simulink model "First_order_integrator_method"  (R2024a)
settings: Solver=VariableStepAuto  StartTime=0.0  StopTime=10.0  RelTol=1e-3
values from neighbouring files (symbols this model uses):
  b = 10    [First_order_parameters.mat]
  k = 400    [First_order_parameters.mat]
  m = 3.6    [First_order_parameters.mat]
settings Model: Creator=nassa  LastModifiedBy=nassa

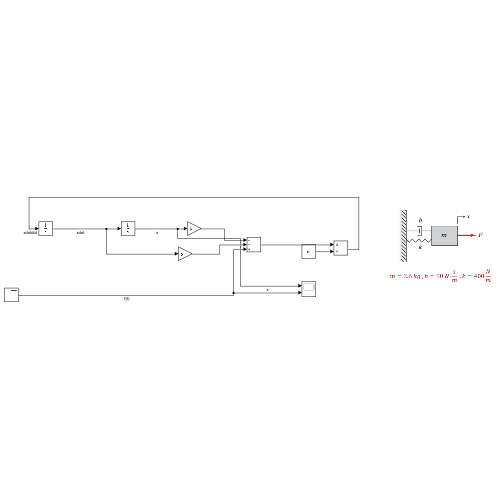
[thumbnail: Simulink's stored preview of the top-level diagram]
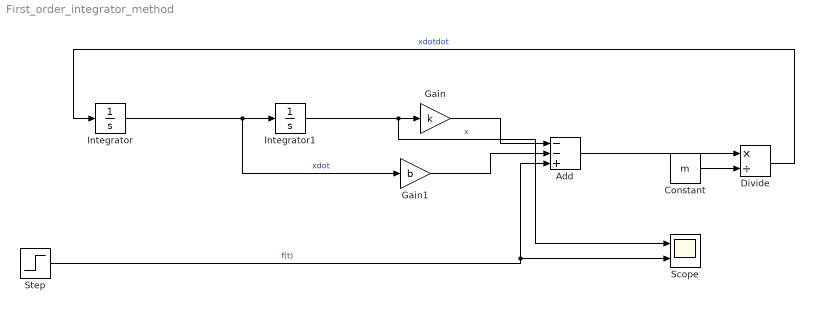
== system First_order_integrator_method ==
  Add : Sum  Inputs=--+
  Constant : Constant  Value=m
  Divide : Product  Inputs=*/
  Gain : Gain  Gain=k
  Gain1 : Gain  Gain=b
  Integrator : Integrator
  Integrator1 : Integrator
  Scope : Scope  NumInputPorts=2
  Step : Step  SampleTime=0
  wires:
  Integrator/1 -> Gain1/1, Integrator1/1  "xdot"
  Integrator1/1 -> Scope/1, Gain/1  "x"
  Divide/1 -> Integrator/1  "xdotdot"
  Gain/1 -> Add/1
  Gain1/1 -> Add/2
  Step/1 -> Scope/2, Add/3  "f(t)"
  Add/1 -> Divide/1
  Constant/1 -> Divide/2
